simulink model "tdeldemo"  (Simulink 6.0)
settings: Solver=VariableStepDiscrete  SolverMode=SingleTasking  StartTime=0  StopTime=11  FixedStep=0.1  MaxStep=0.1  RelTol=1e-3  AbsTol=1e-6
settings Model: Creator=The MathWorks Inc.  LastModifiedBy=batserve  ExtModeTrigMode=oneshot  ExtModeAutoUpdateStatusClock=off
settings DataIOCC: ExternalInput=[]  InitialState=[]  LimitDataPoints=off  SaveOutput=off  TimeSaveName=t
settings OptimizationCC: BooleanDataType=off
settings DebuggingCC: CheckExecutionContextPreStartOutputMsg=on  CheckExecutionContextRuntimeOutputMsg=on  SolverPrmCheckMsg=none
settings HardwareCC: TargetUnknown=on

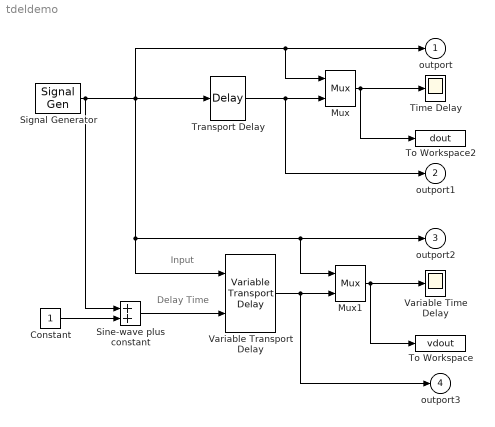
== system tdeldemo ==
  note: Delay Time
  note: Input
  Constant : Constant
  Mux : Mux  Inputs=2
  Mux1 : Mux  Inputs=2
  Signal Generator : SignalGenerator
  Sine-wave plus constant : Sum  SaturateOnIntegerOverflow=on  InputSameDT=on
  Time Delay : Scope
      settings: TickLabels=on  TimeRange=2  YMin=-1  YMax=1  DataFormat=Array
  To Workspace : ToWorkspace  VariableName=vdout  SampleTime=-1  SaveFormat=Array
      settings: MaxDataPoints=10000
  To Workspace2 : ToWorkspace  VariableName=dout  SampleTime=-1  SaveFormat=Array
      settings: MaxDataPoints=10000
  Transport Delay : TransportDelay  DelayTime=0.2
  Variable Transport Delay : VariableTransportDelay  MaximumDelay=3
  Variable Time Delay : Scope
      settings: TickLabels=on  TimeRange=2  YMin=-1  YMax=1  DataFormat=Array
  outport : Outport  InitialOutput=0
  outport1 : Outport  Port=2  InitialOutput=0
  outport2 : Outport  Port=3  InitialOutput=0
  outport3 : Outport  Port=4  InitialOutput=0
  wires:
  Transport Delay/1 -> outport1/1, Mux/2
  Variable Transport Delay/1 -> outport3/1, Mux1/2
  Mux1/1 -> Variable Time Delay/1, To Workspace/1
  Mux/1 -> Time Delay/1, To Workspace2/1
  Sine-wave plus constant/1 -> Variable Transport Delay/2
  Signal Generator/1 -> Sine-wave plus constant/1, outport2/1, Mux1/1, Variable Transport Delay/1, Mux/1, outport/1, Transport Delay/1
  Constant/1 -> Sine-wave plus constant/2
